simulink model "UAV_RefModel"  (R2013a)
settings: Solver=ode3  StartTime=0.0  StopTime=150  FixedStep=SampleTime  RelTol=1e-3
undefined symbols (not defined in the file or in its folder): AC, Earth, Env, IntegerTimeDelay, m, Navigation, Navigation_Lib, OperatingPoint, s, SampleTime, TrimCondition, WGS84
libraries: Sensors_Lib x13, simulink x7, aerolib6dofsys x4, Actuator_Lib x2, aerolibconvert2 x2, aerolibasang x2, aerolibutil x1, aerolibtransform2 x1, Environment_Lib x1, Aero_Lib x1, Propulsion_Lib x1, Gravity_Lib x1
settings Model: Creator=Paul Freeman  LastModifiedBy=descobar
settings DataIOCC: LimitDataPoints=off  SignalLoggingSaveFormat=ModelDataLogs  SaveOutput=off  SignalLogging=off
settings OptimizationCC: ExpressionDepthLimit=2147483647
settings DebuggingCC: FcnCallInpInsideContextMsg=UseLocalSettings  StrictBusMsg=Warning
settings HardwareCC: ProdLargestAtomicInteger=Long  ProdLargestAtomicFloat=Double  ProdIntDivRoundTo=Zero  ProdEndianess=BigEndian  ProdHWDeviceType=Freescale->32-bit PowerPC
settings SFSimCC: SimParseCustomCode=off
settings GRTTargetCC: CombineOutputUpdateFcns=off  GRTInterface=on

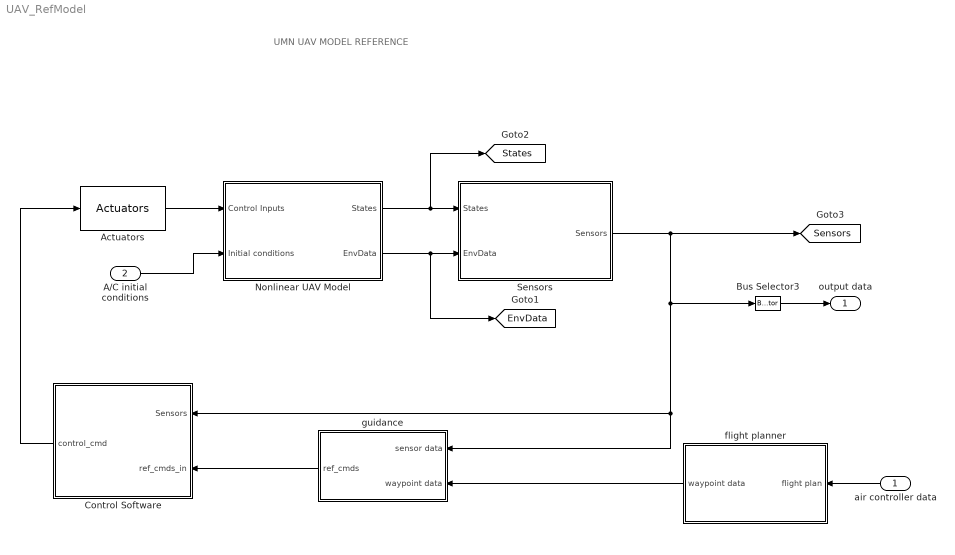
== system UAV_RefModel ==
  note: UMN UAV
      | MODEL REFERENCE
  air controller data : Inport
  A/C initial conditions : Inport  Port=2
  Actuators : Actuator_Lib/Actuators
  Bus Selector3 : BusSelector  OutputSignals=Geodetic Latitude [rad],Geodetic Longitude [rad],Altitude [m],h [m],X_e [m]  OutputAsBus=on
  Control Software : Subsystem
  Nonlinear UAV Model : Subsystem  AncestorBlock=NonlinearModel_Lib/Nonlinear UAV Model
  Sensors : Subsystem  AncestorBlock=Sensors_Lib/Sensors
  flight planner : Subsystem
  "guidance " : Subsystem
  output data : Outport
  tag scope: EnvData=global, Sensors=global, States=global
  wires:
  Sensors/1(Sensors) -> "guidance "/1(sensor data), Control Software/1(Sensors), Bus Selector3/1, [Sensors]
  Nonlinear UAV Model/1(States) -> Sensors/1(States), [States]
  Nonlinear UAV Model/2(EnvData) -> Sensors/2(EnvData), [EnvData]
  Control Software/1(control_cmd) -> Actuators/1
  Actuators/1 -> Nonlinear UAV Model/1(Control Inputs)
  "guidance "/1(ref_cmds) -> Control Software/2(ref_cmds_in)
  flight planner/1(waypoint data) -> "guidance "/2(waypoint data)
  Bus Selector3/1 -> output data/1
  air controller data/1 -> flight planner/1(flight plan)
  A/C initial conditions/1 -> Nonlinear UAV Model/2(Initial conditions)

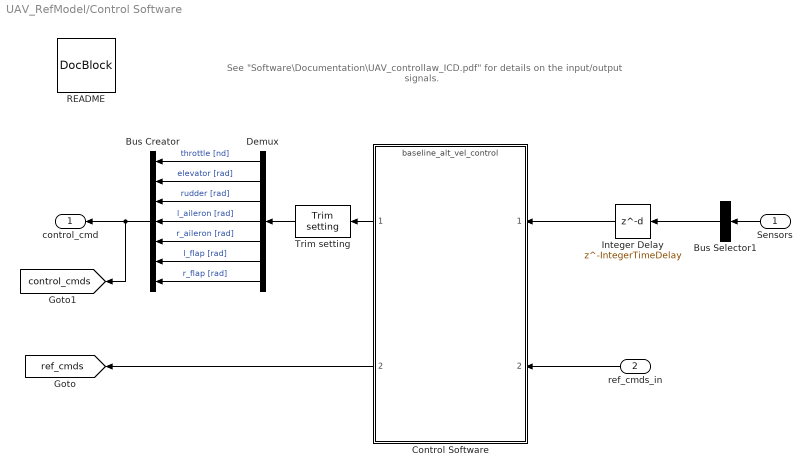
== system UAV_RefModel/Control Software ==
  note: See "Software\Documentation\UAV_controllaw_ICD.pdf" for
      | details on the input/output signals.
  Sensors : Inport
  ref_cmds_in : Inport  Port=2
  Bus Creator : BusCreator  Inputs=7
  Bus Selector1 : BusSelector  OutputSignals=phi [rad],theta [rad],psi [rad],p [rad/s],q [rad/s],r [rad/s],Ax [m/s^2],Ay [m/s^2],Az [m/s^2],h [m],V_s [m/s],alpha [rad],beta [rad],Geodetic Latitude [rad],Geodetic Longitude [rad],Altitude [m],Xdot [m/s],Ydot [m/s],Zdot [m/s]  OutputAsBus=on
  Control Software : ModelReference  ModelNameDialog=baseline_alt_vel_control  Variant=on  ModelReferenceVersion=1.189  CopyOfModelName=baseline_alt_vel_control  DefaultDataLogging=off
  Demux : Demux  Outputs=7
  Integer Delay : Delay  DelayLength=IntegerTimeDelay  InitialCondition=repmat([TrimCondition.AttitudeIni;TrimCondition.RatesIni;TrimCondition.AccelsIni;OperatingPoint.op_report.Outputs(4).y;TrimCondition.WindAxesIni;TrimCondition.LLIni;0; zeros(3,1)],[1,IntegerTimeDelay])  InputProcessing=Inherited
  README : simulink/Model-Wide Utilities/DocBlock  DocumentType=Text
      content=|
      | Control Law Block
      |
      | This block uses Model Referencing to allow the user to easily switch out
      | control law implementations. An example usage would be first a user develops
      | a control law using simulink blocks. This controller is referred to as the
      | "simulink controller" and would be selected by setting the variable
      | "controller_mode" to 2. Once the development is completed, the user then
      | implements the Simulink controller into C-code suitable for integration
      | with the UAV software. This controller is referred to as the "flight code"
      | and would be selected by setting "controller_mode" to 1.
      |
      | This is done using the Simulink.Variant object. See the documentation for
      | more detail. The user can specify any number of variants for the Control
      | Software block; edit the ModelReferenceParameters by right-clicking this
      | block to set which Simulink model is reference for each Variant object.
      | Note that these objects must be present in the base workspace. It
      | is strongly recommended that you use the "simulink_controller.mdl" file as
      | a starting place and "Save As" to a different file name.
      |
      | In summary, to switch the Control Software, modify the "contoller_mode"
      | variable:
      | 1 = flight code controller (C implementation)
      | 2 = simulink controller (empty simulink model)
      |
      |
      | See "Software\Documentation\UAV_controllaw_ICD.pdf" for details on the
      | input/output signals.
      |
      | The control_cmd signal must have the following order:
      | throttle
      | elevator
      | rudder
      | l_aileron
      | r_aileron
      | l_flap
      | r_flap
      |
      | Control Inputs Sign Convention
      | TED = Trailing Edge Down
      | TEL = Trailing Edge Left
      | ------------------------
      | Elevator: +TED
      | Rudder: +TEL
      | Aileron: +TED, da = (da_R-da_L)/2
      | Throttle: always positive
      | Flap: +TED
      |
      |
      | The refrence command signal must have the following order:
      | 1. phi_cmd
      | 2. theta_cmd
      | 3. psi_cmd
      | 4. p_cmd
      | 5. q_cmd
      | 6. r_cmd
      | 7. V_s_cmd
      | 8. h_cmd
      | 9. gndtrk_cmd
      | 10. aoa_cmd
      | 11. aos_cmd
      | 12. gamma_cmd
      | Note the trimmed value of pitch angle theta is included in the reference
      | command. Use the Doublet Generator block (or other signal generating block)
      | to input reference commands to the Control Software.
  "Trim setting " : Actuator_Lib/Trim setting 
  control_cmd : Outport
  tag scope: control_cmds=global, ref_cmds=global
  wires:
  Control Software/1 -> "Trim setting "/1
  Sensors/1 -> Bus Selector1/1
  ref_cmds_in/1 -> Control Software/2
  Bus Creator/1 -> control_cmd/1, [control_cmds]
  Demux/1 -> Bus Creator/1  "throttle [nd]"
  Demux/2 -> Bus Creator/2  "elevator [rad]"
  Demux/3 -> Bus Creator/3  "rudder [rad]"
  Demux/4 -> Bus Creator/4  "l_aileron [rad]"
  Demux/5 -> Bus Creator/5  "r_aileron [rad]"
  Demux/6 -> Bus Creator/6  "l_flap [rad]"
  Demux/7 -> Bus Creator/7  "r_flap [rad]"
  Integer Delay/1 -> Control Software/1
  Bus Selector1/1 -> Integer Delay/1
  "Trim setting "/1 -> Demux/1
  Control Software/2 -> [ref_cmds]

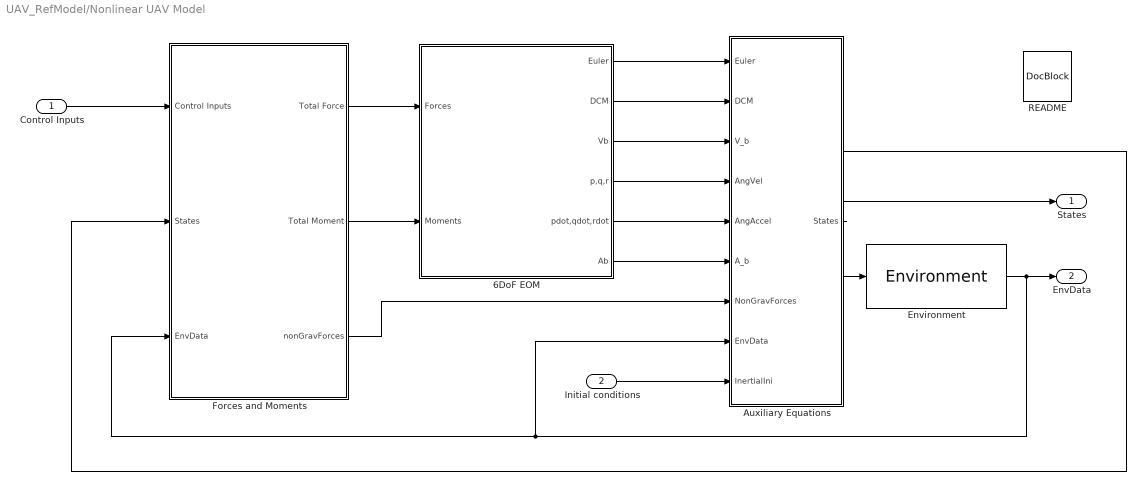
== system UAV_RefModel/Nonlinear UAV Model ==
  Control Inputs : Inport
  Initial conditions : Inport  Port=2
  6DoF EOM : Subsystem  mask(6DoF EoM (Body Axis)){units=Metric (MKS), mtype=Fixed, rep=Euler Angles, xme_0=TrimCondition.InertialIni, Vm_0=TrimCondition.VelocitiesIni, eul_0=TrimCondition.AttitudeIni, pm_0=TrimCondition.RatesIni, mass_0=AC.Mass, mass_e=0.5, mass_f=2.0, inertia=AC.Inertia.Matrix, inertia_e=eye(3), inertia_f=2*eye(3), k_quat=1.0}
      mask prompts: mtype "Mass type:"; rep "Representation:"; xme_0 "Initial position in inertial axes [Xe,Ye,Ze]:"; Vm_0 "Initial velocity in body axes [U,v,w]:"; eul_0 "Initial Euler orientation [roll, pitch, yaw]:"; pm_0 "Initial body rotation rates [p,q,r]:"; mass_0 "Initial mass:"; mass_e "Empty mass:"; mass_f "Full mass:"; inertia_e "Empty inertia matrix:"; inertia_f "Full inertia matrix:"; k_quat "Gain for quaternion normalization:"
      mask help:
      | Integrate the six-degrees-of-freedom equations of motion in body axis.
      |
      | This block has been modified from the original Aerospace Blockset
      | implementation. The inertial position vector (Xe) is no longer computed.
      | The original block did not have a way to add steady state winds to the
      | inertial velocities (Ve) prior to integrating to get Xe. Therefore, this
      | step is performed in the Auxiliary Equations block.
      mask Help: eval('asbhelp(''sixdof_euler_angles'')');
      mask TypeOptions units: Metric (MKS) | English (Velocity in ft/s) | English (Velocity in kts)
      mask TypeOptions mtype: Fixed | Simple Variable | Custom Variable
      mask Callback mtype: aeroicon('aeroblk6dofbody');
      mask TypeOptions rep: Euler Angles | Quaternion
      mask Callback rep: aeroicon('aeroblk6dofbody');
  Auxiliary Equations : Subsystem  AncestorBlock=AuxEq_Lib/Auxiliary Equations
  Environment : Environment_Lib/Environment
  Forces and Moments : Subsystem
  README : simulink/Model-Wide Utilities/DocBlock  DocumentType=Text
      content=|
      | Nonlinear UAV Model
      |
      | This block implements the nonlinear UAV dynamics model. Beginning on the
      | left, the Forces and Moments block models all of the relevant external
      | forces and moments acting on the aircraft.
      |
      | The 6DoF EOM block implements the six degree of freedom, fixed mass,
      | flat, non-rotating Earth, rigid body equations of motion. This block has
      | been modified from the original Aerospace Blockset implementation. The
      | inertial position vector (Xe) is no longer computed. The original block
      | did not have a way to add steady state winds to the inertial velocities
      | (Ve) prior to integrating to get Xe. Therefore, this step is performed in
      | the Auxiliary Equations block.
      |
      | The Auxiliary Equations computes other relevant variables (such as angle
      | of attack, indicated airspeed, etc) from state data. In this block are
      | the Navigation equations.
      |
      | Finally, the Environment block has Aerospace Blockset models for Earth's
      | atmosphere, gravity, and magnetic fields. Winds are modeled in two
      | portions: steady and unsteady. The steady portion is defined by a speed
      | and direction, and is horizontal only. The unsteady portion is made up of
      | a wind shear model and a turbulence model.
  States : Outport
  EnvData : Outport  Port=2
  wires:
  6DoF EOM/6(Ab) -> Auxiliary Equations/6(A_b)
  6DoF EOM/5(pdot,qdot,rdot) -> Auxiliary Equations/5(AngAccel)
  6DoF EOM/4(p,q,r) -> Auxiliary Equations/4(AngVel)
  6DoF EOM/3(Vb) -> Auxiliary Equations/3(V_b)
  6DoF EOM/2(DCM) -> Auxiliary Equations/2(DCM)
  6DoF EOM/1(Euler) -> Auxiliary Equations/1(Euler)
  Control Inputs/1 -> Forces and Moments/1(Control Inputs)
  Forces and Moments/1(Total Force) -> 6DoF EOM/1(Forces)
  Forces and Moments/2(Total Moment) -> 6DoF EOM/2(Moments)
  Auxiliary Equations/1(States) -> States/1, Forces and Moments/2(States), Environment/1
  Forces and Moments/3(nonGravForces) -> Auxiliary Equations/7(NonGravForces)
  Environment/1 -> Forces and Moments/3(EnvData), Auxiliary Equations/8(EnvData), EnvData/1
  Initial conditions/1 -> Auxiliary Equations/9(InertialIni)

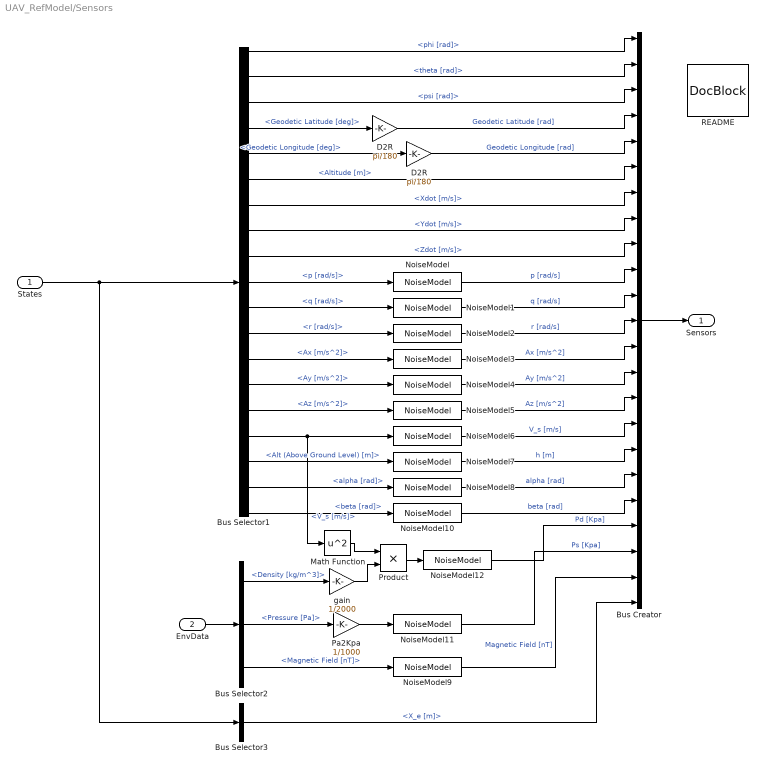
== system UAV_RefModel/Sensors ==
  States : Inport
  EnvData : Inport  Port=2
  Bus Creator : BusCreator  Inputs=23
  Bus Selector1 : BusSelector  OutputSignals=Euler [rad].phi [rad],Euler [rad].theta [rad],Euler [rad].psi [rad],Nav.Geodetic Latitude [deg],Nav.Geodetic Longitude [deg],Nav.Altitude [m],V_e [m/s].Xdot [m/s],V_e [m/s].Ydot [m/s],V_e [m/s].Zdot [m/s],AngVel [rad/s].p [rad/s],AngVel [rad/s].q [rad/s],AngVel [rad/s].r [rad/s],Accels [m/s^2].Ax [m/s^2],Accels [m/s^2].Ay [m/s^2],Accels [m/s^2].Az [m/s^2],WindAxesParam.V_s [m/s],Nav.Alt (Above Ground Level) [m],WindAxesParam.alpha [rad],WindAxesParam.beta [rad]
  Bus Selector2 : BusSelector  OutputSignals=Density [kg/m^3],Pressure [Pa],Magnetic Field [nT]
  Bus Selector3 : BusSelector  OutputSignals=X_e [m]
  D2R : Gain  Gain=pi/180  SampleTime=SampleTime
  "D2R " : Gain  Gain=pi/180  SampleTime=SampleTime
  Math Function : Math  Operator=square  SaturateOnIntegerOverflow=on
  NoiseModel : Sensors_Lib/NoiseModel  noise_on=AC.Sensors.NoiseOn  sigma=AC.Sensors.IMU.p_noise  seed=878230  bias=AC.Sensors.IMU.p_bias  scf=AC.Sensors.IMU.p_scf  timestep=SampleTime
  NoiseModel1 : Sensors_Lib/NoiseModel  noise_on=AC.Sensors.NoiseOn  sigma=AC.Sensors.IMU.q_noise  seed=878231  bias=AC.Sensors.IMU.q_bias  scf=AC.Sensors.IMU.q_scf  timestep=SampleTime
  NoiseModel10 : Sensors_Lib/NoiseModel  noise_on=AC.Sensors.NoiseOn  sigma=AC.Sensors.AirData.beta_noise  seed=87828  bias=AC.Sensors.AirData.beta_bias  scf=AC.Sensors.AirData.beta_scf  timestep=SampleTime
  NoiseModel11 : Sensors_Lib/NoiseModel  noise_on=AC.Sensors.NoiseOn  sigma=AC.Sensors.AirData.Ps_noise  seed=8782378  bias=AC.Sensors.AirData.Ps_bias  scf=AC.Sensors.AirData.Ps_scf  timestep=SampleTime
  NoiseModel12 : Sensors_Lib/NoiseModel  noise_on=AC.Sensors.NoiseOn  sigma=AC.Sensors.AirData.Pd_noise  seed=87823  bias=AC.Sensors.AirData.Pd_bias  scf=AC.Sensors.AirData.Pd_scf  timestep=SampleTime
  NoiseModel2 : Sensors_Lib/NoiseModel  noise_on=AC.Sensors.NoiseOn  sigma=AC.Sensors.IMU.r_noise  seed=878232  bias=AC.Sensors.IMU.r_bias  scf=AC.Sensors.IMU.r_scf  timestep=SampleTime
  NoiseModel3 : Sensors_Lib/NoiseModel  noise_on=AC.Sensors.NoiseOn  sigma=AC.Sensors.IMU.ax_noise  seed=878233  bias=AC.Sensors.IMU.ax_bias  scf=AC.Sensors.IMU.ax_scf  timestep=SampleTime
  NoiseModel4 : Sensors_Lib/NoiseModel  noise_on=AC.Sensors.NoiseOn  sigma=AC.Sensors.IMU.ay_noise  seed=878234  bias=AC.Sensors.IMU.ay_bias  scf=AC.Sensors.IMU.ay_scf  timestep=SampleTime
  NoiseModel5 : Sensors_Lib/NoiseModel  noise_on=AC.Sensors.NoiseOn  sigma=AC.Sensors.IMU.az_noise  seed=878235  bias=AC.Sensors.IMU.az_bias  scf=AC.Sensors.IMU.az_scf  timestep=SampleTime
  NoiseModel6 : Sensors_Lib/NoiseModel  noise_on=AC.Sensors.NoiseOn  sigma=AC.Sensors.AirData.ias_noise  seed=878236  bias=AC.Sensors.AirData.ias_bias  scf=AC.Sensors.AirData.ias_scf  timestep=SampleTime
  NoiseModel7 : Sensors_Lib/NoiseModel  noise_on=AC.Sensors.NoiseOn  sigma=AC.Sensors.AirData.h_noise  seed=87828  bias=AC.Sensors.AirData.h_bias  scf=AC.Sensors.AirData.h_scf  timestep=SampleTime
  NoiseModel8 : Sensors_Lib/NoiseModel  noise_on=AC.Sensors.NoiseOn  sigma=AC.Sensors.AirData.alpha_noise  seed=87828  bias=AC.Sensors.AirData.alpha_bias  scf=AC.Sensors.AirData.alpha_scf  timestep=SampleTime
  NoiseModel9 : Sensors_Lib/NoiseModel  noise_on=AC.Sensors.NoiseOn  sigma=[AC.Sensors.IMU.hx_noise, AC.Sensors.IMU.hy_noise,AC.Sensors.IMU.hz_noise]  seed=878237  bias=[AC.Sensors.IMU.hx_bias, AC.Sensors.IMU.hy_bias, AC.Sensors.IMU.hz_bias]  scf=[AC.Sensors.IMU.hx_scf, AC.Sensors.IMU.hy_scf, AC.Sensors.IMU.hz_scf]  timestep=SampleTime
  Pa2Kpa : Gain  Gain=1/1000
  Product : Product  RndMeth=Zero
  README : simulink/Model-Wide Utilities/DocBlock  DocumentType=Text
      content=|
      | Sensors
      |
      | This block implements sensor models on selected signals. A generic block
      | is used that applies a bias, scale factor, and band limited white noise to
      | a given signal. The parameters for each block are stored in the aircraft
      | configuration data structure (AC):
      |
      | >> AC.Sensors
      |
      | ans =
      |
      |     NoiseOn: 1
      |         IMU: [1x1 struct]
      |     AirData: [1x1 struct]
      |
      | Note the "NoiseOn" boolean flag- by setting this flag to zero, the sensor
      | model will be disabled.
      |
      | Currently, the bias and scale factor errors are not used; only white noise
      | is applied.
  gain : Gain  Gain=1/2000
  Sensors : Outport
  wires:
  Bus Selector1/15 -> NoiseModel5/1  "<Az [m/s^2]>"
  Bus Selector1/14 -> NoiseModel4/1  "<Ay [m/s^2]>"
  Bus Selector1/13 -> NoiseModel3/1  "<Ax [m/s^2]>"
  Bus Selector1/12 -> NoiseModel2/1  "<r [rad/s]>"
  Bus Selector1/11 -> NoiseModel1/1  "<q [rad/s]>"
  Bus Selector1/10 -> NoiseModel/1  "<p [rad/s]>"
  States/1 -> Bus Selector3/1, Bus Selector1/1
  Bus Selector1/16 -> NoiseModel6/1, Math Function/1  "<V_s [m/s]>"
  Bus Selector2/3 -> NoiseModel9/1  "<Magnetic Field [nT]>"
  Bus Selector1/17 -> NoiseModel7/1  "<Alt (Above Ground Level) [m]>"
  EnvData/1 -> Bus Selector2/1
  Bus Selector1/18 -> NoiseModel8/1  "<alpha [rad]>"
  Bus Selector1/19 -> NoiseModel10/1  "<beta [rad]>"
  Bus Selector2/2 -> Pa2Kpa/1  "<Pressure [Pa]>"
  Pa2Kpa/1 -> NoiseModel11/1
  Bus Selector2/1 -> gain/1  "<Density [kg/m^3]>"
  Math Function/1 -> Product/1
  gain/1 -> Product/2
  Product/1 -> NoiseModel12/1
  Bus Creator/1 -> Sensors/1
  Bus Selector1/1 -> Bus Creator/1  "<phi [rad]>"
  Bus Selector1/2 -> Bus Creator/2  "<theta [rad]>"
  Bus Selector1/3 -> Bus Creator/3  "<psi [rad]>"
  Bus Selector1/4 -> D2R/1  "<Geodetic Latitude [deg]>"
  Bus Selector1/5 -> "D2R "/1  "<Geodetic Longitude [deg]>"
  Bus Selector1/6 -> Bus Creator/6  "<Altitude [m]>"
  Bus Selector1/7 -> Bus Creator/7  "<Xdot [m/s]>"
  Bus Selector1/8 -> Bus Creator/8  "<Ydot [m/s]>"
  Bus Selector1/9 -> Bus Creator/9  "<Zdot [m/s]>"
  NoiseModel/1 -> Bus Creator/10  "p [rad/s]"
  NoiseModel1/1 -> Bus Creator/11  "q [rad/s]"
  NoiseModel2/1 -> Bus Creator/12  "r [rad/s]"
  NoiseModel3/1 -> Bus Creator/13  "Ax [m/s^2]"
  NoiseModel4/1 -> Bus Creator/14  "Ay [m/s^2]"
  NoiseModel5/1 -> Bus Creator/15  "Az [m/s^2]"
  NoiseModel6/1 -> Bus Creator/16  "V_s [m/s]"
  NoiseModel7/1 -> Bus Creator/17  "h [m]"
  NoiseModel8/1 -> Bus Creator/18  "alpha [rad]"
  NoiseModel10/1 -> Bus Creator/19  "beta [rad]"
  NoiseModel12/1 -> Bus Creator/20  "Pd [Kpa]"
  NoiseModel11/1 -> Bus Creator/21  "Ps [Kpa]"
  NoiseModel9/1 -> Bus Creator/22  "Magnetic Field [nT]"
  D2R/1 -> Bus Creator/4  "Geodetic Latitude [rad]"
  "D2R "/1 -> Bus Creator/5  "Geodetic Longitude [rad]"
  Bus Selector3/1 -> Bus Creator/23  "<X_e [m]>"

== system UAV_RefModel/flight planner ==
  flight plan : Inport
  Bus Creator : BusCreator  Inputs=2
  Waypoint generator : MATLAB Function  TreatAsAtomicUnit=on
  waypoint data : Outport
  wires:
  Waypoint generator/1(waypoint) -> Bus Creator/1
  Waypoint generator/2(nPoints) -> Bus Creator/2
  Bus Creator/1 -> waypoint data/1
  flight plan/1 -> Waypoint generator/1(plan)

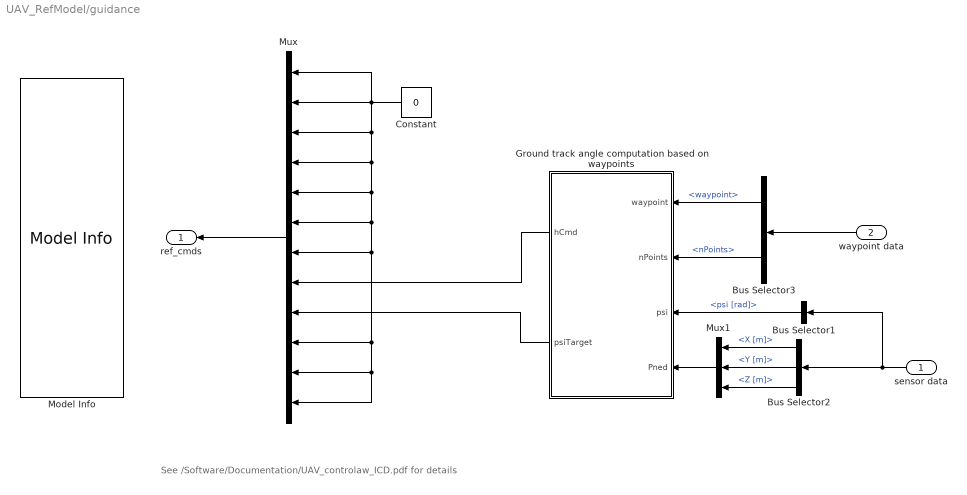
== system UAV_RefModel/guidance  ==
  note: See /Software/Documentation/UAV_controlaw_ICD.pdf
      | for details
  sensor data : Inport
  waypoint data : Inport  Port=2
  Bus Selector1 : BusSelector  OutputSignals=psi [rad]
  Bus Selector2 : BusSelector  OutputSignals=X_e [m].X [m],X_e [m].Y [m],X_e [m].Z [m]
  Bus Selector3 : BusSelector  OutputSignals=waypoint,nPoints
  Constant : Constant  Value=0
  Ground track angle computation based on waypoints : MATLAB Function  TreatAsAtomicUnit=on
  Model Info : simulink/Model-Wide Utilities/Model Info  InitialBlockCM=None  BlockCM=None  Frame=on  DisplayStringWithTags=|  HorizontalTextAlignment=Center  LeftAlignmentValue=0.5  SourceBlockDiagram=UAV_RefModel  TagMaxNumber=20
      | Ref Cmd Port Info
      | 
      | 1. phi_cmd
      | 2. theta_cmd
      | 3. psi_cmd
      | 4. p_cmd
      | 5. q_cmd
      | 6. r_cmd
      | 7. V_s_cmd
      | 8. h_cmd
      | 9. gndtrk_cmd
      | 10. aoa_cmd
      | 11. aos_cmd
      | 12. gamma_cmd
  Mux : Mux  Inputs=12
  Mux1 : Mux  Inputs=3
  ref_cmds : Outport
  wires:
  Mux/1 -> ref_cmds/1
  Bus Selector2/1 -> Mux1/1  "<X [m]>"
  Bus Selector2/2 -> Mux1/2  "<Y [m]>"
  Bus Selector2/3 -> Mux1/3  "<Z [m]>"
  sensor data/1 -> Bus Selector1/1, Bus Selector2/1
  Bus Selector1/1 -> Ground track angle computation based on waypoints/3(psi)  "<psi [rad]>"
  Mux1/1 -> Ground track angle computation based on waypoints/4(Pned)
  Bus Selector3/1 -> Ground track angle computation based on waypoints/1(waypoint)  "<waypoint>"
  Bus Selector3/2 -> Ground track angle computation based on waypoints/2(nPoints)  "<nPoints>"
  Ground track angle computation based on waypoints/2(psiTarget) -> Mux/9
  Constant/1 -> Mux/3, Mux/4, Mux/5, Mux/6, Mux/7, Mux/10, Mux/11, Mux/12, Mux/1, Mux/2
  waypoint data/1 -> Bus Selector3/1
  Ground track angle computation based on waypoints/1(hCmd) -> Mux/8

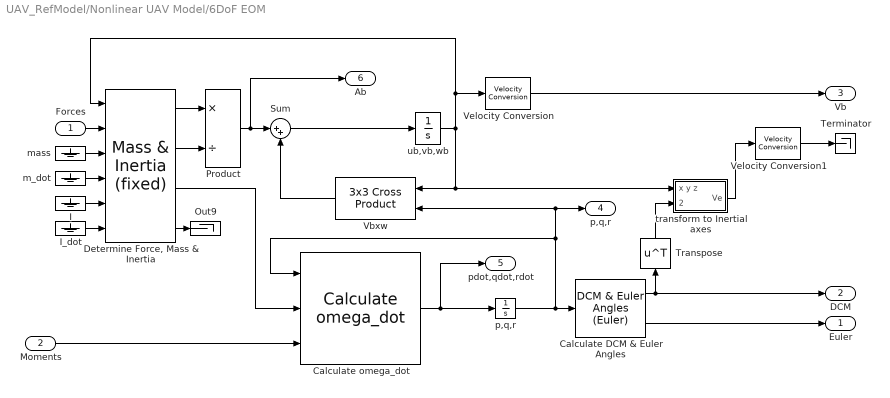
== system UAV_RefModel/Nonlinear UAV Model/6DoF EOM ==
  Forces : Inport
  Moments : Inport  Port=2
  Calculate DCM & Euler Angles : aerolib6dofsys/DCM & Euler Angles (Euler)  SystemSampleTime=-1
  Calculate omega_dot : aerolib6dofsys/Calculate omega_dot
  "Determine Force, Mass & Inertia" : aerolib6dofsys/Mass & Inertia (fixed)  SystemSampleTime=-1
  I : Ground
  I_dot : Ground
  Out9 : Terminator
  Product : Product  Inputs=*/  SaturateOnIntegerOverflow=on  OutDataTypeStr=Inherit: Same as first input
  Sum : Sum  Inputs=|++  SaturateOnIntegerOverflow=on
  Terminator : Terminator
  Transpose : Math  Operator=transpose  SaturateOnIntegerOverflow=on
  Vbxw : aerolibutil/3x3 Cross Product
  Velocity Conversion : aerolibconvert2/Velocity Conversion  IU=m/s  OU=m/s
  Velocity Conversion1 : aerolibconvert2/Velocity Conversion  IU=m/s  OU=m/s
  m_dot : Ground
  mass : Ground
  "p,q,r " : Integrator  InitialCondition=pm_0
  "transform to Inertial axes " : Subsystem  mask(Vector Transformation){}
      mask Display: disp('L_EB')
  ub,vb,wb : Integrator  InitialCondition=convvel(Vm_0,'m/s','m/s')
  Euler : Outport
  DCM : Outport  Port=2
  Vb : Outport  Port=3
  p,q,r : Outport  Port=4
  pdot,qdot,rdot : Outport  Port=5
  Ab : Outport  Port=6
  wires:
  Velocity Conversion1/1 -> Terminator/1
  Velocity Conversion/1 -> Vb/1
  "Determine Force, Mass & Inertia"/3 -> Calculate omega_dot/2
  Calculate DCM & Euler Angles/2 -> Euler/1
  Vbxw/1 -> Sum/2
  ub,vb,wb/1 -> Velocity Conversion/1, "Determine Force, Mass & Inertia"/1, "transform to Inertial axes "/1(x y z), Vbxw/1
  Sum/1 -> ub,vb,wb/1
  "transform to Inertial axes "/1(Ve) -> Velocity Conversion1/1
  "p,q,r "/1 -> Calculate omega_dot/1, p,q,r/1, Vbxw/2, Calculate DCM & Euler Angles/1
  Moments/1 -> Calculate omega_dot/3
  Forces/1 -> "Determine Force, Mass & Inertia"/2
  Product/1 -> Sum/1, Ab/1
  Calculate DCM & Euler Angles/1 -> DCM/1, Transpose/1
  Transpose/1 -> "transform to Inertial axes "/2(transform coefficients)
  mass/1 -> "Determine Force, Mass & Inertia"/3
  "Determine Force, Mass & Inertia"/2 -> Product/2
  m_dot/1 -> "Determine Force, Mass & Inertia"/4
  "Determine Force, Mass & Inertia"/4 -> Out9/1
  Calculate omega_dot/1 -> pdot,qdot,rdot/1, "p,q,r "/1
  I/1 -> "Determine Force, Mass & Inertia"/5
  I_dot/1 -> "Determine Force, Mass & Inertia"/6
  "Determine Force, Mass & Inertia"/1 -> Product/1

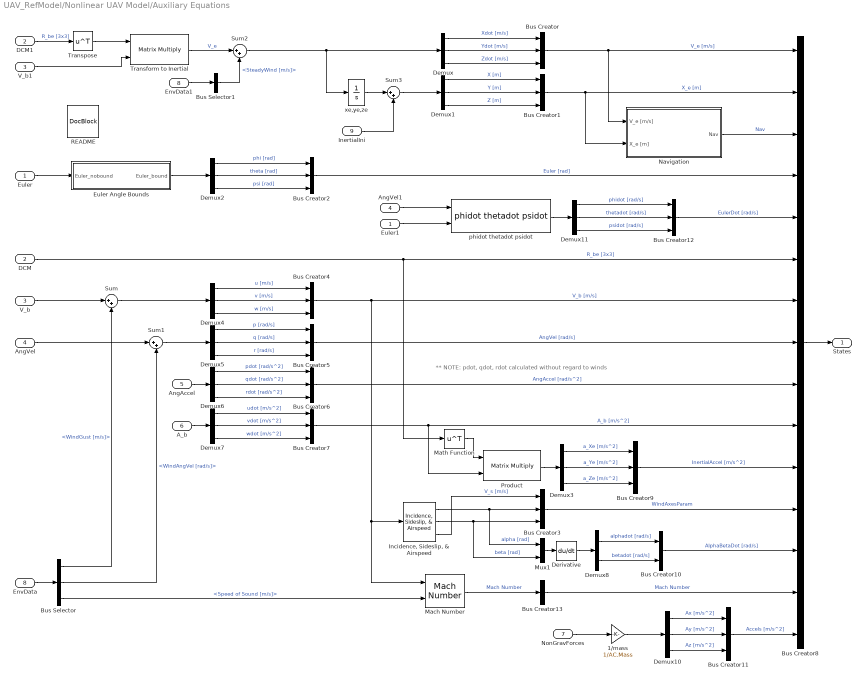
== system UAV_RefModel/Nonlinear UAV Model/Auxiliary Equations ==
  note: ** NOTE: pdot, qdot, rdot calculated without regard to winds
  Euler : Inport
  DCM : Inport  Port=2
  V_b : Inport  Port=3
  AngVel : Inport  Port=4
  AngAccel : Inport  Port=5
  A_b : Inport  Port=6
  NonGravForces : Inport  Port=7
  EnvData : Inport  Port=8
  InertialIni : Inport  Port=9
  1/mass : Gain  Gain=1/AC.Mass
  AngVel1 : InportShadow  Port=4
  Bus Creator{,1..7,9,11..12} (11 alike) : BusCreator  Inputs=3
  Bus Creator10 : BusCreator  Inputs=2
  Bus Creator13 : BusCreator  Inputs=1
  Bus Creator8 : BusCreator  Inputs=15
  Bus Selector : BusSelector  OutputSignals=WindGust [m/s],WindAngVel [rad/s],Speed of Sound [m/s]
  Bus Selector1 : BusSelector  OutputSignals=SteadyWind [m/s]
  DCM1 : InportShadow  Port=2
  Demux{,1..7,10..11} (10 alike) : Demux  Outputs=3
  Demux8 : Demux  Outputs=2
  Derivative : Derivative
  EnvData1 : InportShadow  Port=8
  Euler Angle Bounds : Subsystem
  Euler1 : InportShadow
  "Incidence, Sideslip, & Airspeed" : aerolibasang/Incidence, Sideslip, & Airspeed
  Mach Number : aerolibasang/Mach Number
  Math Function : Math  Operator=transpose  SaturateOnIntegerOverflow=on
  Mux1 : Mux  Inputs=2
  Navigation : Subsystem  Description=|  AncestorBlock=Navigation_Lib/Navigation
      | This model produces the followng navigation data for the UAV flight:
      |                                                                     
      | * Geodetic Latitude                                                 
      | * Geodetic Longitude                                                
      | * Geodetic Altitude                                                 
      | * Altitude above Mean Sea Level                                     
      | * Gravitational acceleration vector
  Product : Product  Multiplication=Matrix(*)  RndMeth=Zero
  README : simulink/Model-Wide Utilities/DocBlock  DocumentType=Text
      content=|
      | Auxiliary Equations
      |
      | This block computes other relevant variables (such as angle of attack,
      | indicated airspeed, etc) from state data. Part of this block is simply to
      | assign signals name and create the States bus.
      |
      | Working from the top of the block downwards:
      |
      | The inertial velocity, V_e, is computed by using the Direction Cosine
      | Matrix (DCM) to transform the body-axis velocities (u,v,w) to the
      | inertial frame. The steady state winds are then added, and the result is
      | V_e. This is integrated to obtain the inertial position, X_e.  The
      | initial condition of the X_e integrator is set by
      | TrimCondition.InertialIni. V_e and X_e are inputs to the Navigation
      | block- see that blocks README for details.
      |
      | Euler angles are bounded by +\- [pi/2, pi, 2*pi] respectively. The time
      | derivatives of the Euler angles are computed using the body-axis rates
      | and the Euler angles.
      |
      | The DCM is included in the States bus as "R_be [3x3]".
      |
      | Body axis velocites and rates, and their derivatives are included. The
      | unsteady (turbulence and gusts) winds are added to the body axis
      | velocities and rates.
      |
      | Inertial accelerations are computed by transforming the body-axis
      | accelerations with the DCM. This step is simplified since we are using a
      | non-rotating Earth.
      |
      | WindAxesParam is the true airspeed, angle of attack, and sideslip angle.
      | The derivatives of alpha and beta are computed using a deriative block.
      | Mach number is simply the ratio between true airspeed and the speed of
      | sound.
      |
      | Accels [m/s^2] is what an accelerometer would read onboard the aircraft.
      |
      | *Note on winds: dividing the wind components into steady and unsteady
      | components is necessary because we do not use an intermediate atmospheric
      | reference frame to account for the motion of the air mass relative to the
      | Earth. We can approximate the physical effects of wind without an
      | additional reference frame by splitting the wind into steady and unsteady
      | components, where the steady component is added to the inertial
      | velocities and the unsteady component is added to the body-axis
      | velocities allows us to
  Sum{,1..3} (4 alike) : Sum  Inputs=|++
  Transform to Inertial : Product  Multiplication=Matrix(*)  RndMeth=Zero
  Transpose : Math  Operator=transpose  SaturateOnIntegerOverflow=on
  V_b1 : InportShadow  Port=3
  phidot thetadot psidot : aerolib6dofsys/DCM & Euler Angles (Euler)/phidot thetadot psidot
  xe,ye,ze : Integrator  InitialCondition=TrimCondition.InertialIni
  States : Outport
  wires:
  Mach Number/1 -> Bus Creator13/1  "Mach Number"
  Demux8/2 -> Bus Creator10/2  "betadot [rad/s]"
  Demux8/1 -> Bus Creator10/1  "alphadot [rad/s]"
  Bus Creator10/1 -> Bus Creator8/13  "AlphaBetaDot [rad/s]"
  Derivative/1 -> Demux8/1
  Mux1/1 -> Derivative/1
  "Incidence, Sideslip, & Airspeed"/3 -> Bus Creator3/1  "V_s [m/s]"
  "Incidence, Sideslip, & Airspeed"/2 -> Mux1/2, Bus Creator3/3  "beta [rad]"
  "Incidence, Sideslip, & Airspeed"/1 -> Mux1/1, Bus Creator3/2  "alpha [rad]"
  Bus Creator8/1 -> States/1
  Navigation/1(Nav) -> Bus Creator8/3  "Nav"
  Bus Creator11/1 -> Bus Creator8/15  "Accels [m/s^2]"
  Euler1/1 -> phidot thetadot psidot/2
  AngVel1/1 -> phidot thetadot psidot/1
  Bus Selector/1 -> Sum/2  "<WindGust [m/s]>"
  Bus Selector/2 -> Sum1/2  "<WindAngVel [rad/s]>"
  Bus Creator9/1 -> Bus Creator8/11  "InertialAccel [m/s^2]"
  Demux3/2 -> Bus Creator9/2  "a_Ye [m/s^2]"
  Demux3/3 -> Bus Creator9/3  "a_Ze [m/s^2]"
  Demux3/1 -> Bus Creator9/1  "a_Xe [m/s^2]"
  Product/1 -> Demux3/1
  Math Function/1 -> Product/1
  V_b/1 -> Sum/1
  AngVel/1 -> Sum1/1
  Sum/1 -> Demux4/1
  Sum1/1 -> Demux5/1
  Bus Selector/3 -> Mach Number/2  "<Speed of Sound [m/s]>"
  EnvData/1 -> Bus Selector/1
  Bus Creator13/1 -> Bus Creator8/14  "Mach Number"
  Bus Creator3/1 -> Bus Creator8/12  "WindAxesParam"
  A_b/1 -> Demux7/1
  Demux7/3 -> Bus Creator7/3  "wdot [m/s^2]"
  Demux7/2 -> Bus Creator7/2  "vdot [m/s^2]"
  Demux7/1 -> Bus Creator7/1  "udot [m/s^2]"
  Bus Creator7/1 -> Bus Creator8/10, Product/2  "A_b [m/s^2]"
  AngAccel/1 -> Demux6/1
  Demux6/3 -> Bus Creator6/3  "rdot [rad/s^2]"
  Demux6/2 -> Bus Creator6/2  "qdot [rad/s^2]"
  Demux6/1 -> Bus Creator6/1  "pdot [rad/s^2]"
  Bus Creator6/1 -> Bus Creator8/9  "AngAccel [rad/s^2]"
  Demux5/3 -> Bus Creator5/3  "r [rad/s]"
  Demux5/2 -> Bus Creator5/2  "q [rad/s]"
  Demux5/1 -> Bus Creator5/1  "p [rad/s]"
  Bus Creator5/1 -> Bus Creator8/8  "AngVel [rad/s]"
  Demux4/3 -> Bus Creator4/3  "w [m/s]"
  Demux4/2 -> Bus Creator4/2  "v [m/s]"
  Demux4/1 -> Bus Creator4/1  "u [m/s]"
  Bus Creator4/1 -> Mach Number/1, "Incidence, Sideslip, & Airspeed"/1, Bus Creator8/7  "V_b [m/s]"
  DCM/1 -> Bus Creator8/6, Math Function/1  "R_be [3x3]"
  Demux2/3 -> Bus Creator2/3  "psi [rad]"
  Demux2/2 -> Bus Creator2/2  "theta [rad]"
  Demux2/1 -> Bus Creator2/1  "phi [rad]"
  Bus Creator2/1 -> Bus Creator8/4  "Euler [rad]"
  Demux1/3 -> Bus Creator1/3  "Z [m]"
  Demux1/2 -> Bus Creator1/2  "Y [m]"
  Demux1/1 -> Bus Creator1/1  "X [m]"
  Bus Creator1/1 -> Bus Creator8/2, Navigation/2(X_e [m])  "X_e [m]"
  Demux/3 -> Bus Creator/3  "Zdot [m/s]"
  Demux/2 -> Bus Creator/2  "Ydot [m/s]"
  Demux/1 -> Bus Creator/1  "Xdot [m/s]"
  Bus Creator/1 -> Bus Creator8/1, Navigation/1(V_e [m/s])  "V_e [m/s]"
  NonGravForces/1 -> 1/mass/1
  1/mass/1 -> Demux10/1
  Demux10/1 -> Bus Creator11/1  "Ax [m/s^2]"
  Demux10/2 -> Bus Creator11/2  "Ay [m/s^2]"
  Demux10/3 -> Bus Creator11/3  "Az [m/s^2]"
  Demux11/3 -> Bus Creator12/3  "psidot [rad/s]"
  Demux11/2 -> Bus Creator12/2  "thetadot [rad/s]"
  Demux11/1 -> Bus Creator12/1  "phidot [rad/s]"
  Bus Creator12/1 -> Bus Creator8/5  "EulerDot [rad/s]"
  phidot thetadot psidot/1 -> Demux11/1
  Transpose/1 -> Transform to Inertial/1
  DCM1/1 -> Transpose/1  "R_be [3x3]"
  EnvData1/1 -> Bus Selector1/1
  Transform to Inertial/1 -> Sum2/1  "V_e"
  Bus Selector1/1 -> Sum2/2  "<SteadyWind [m/s]>"
  Sum2/1 -> Demux/1, xe,ye,ze/1
  V_b1/1 -> Transform to Inertial/2
  Euler/1 -> Euler Angle Bounds/1(Euler_nobound)
  Euler Angle Bounds/1(Euler_bound) -> Demux2/1
  Sum3/1 -> Demux1/1
  xe,ye,ze/1 -> Sum3/1
  InertialIni/1 -> Sum3/2

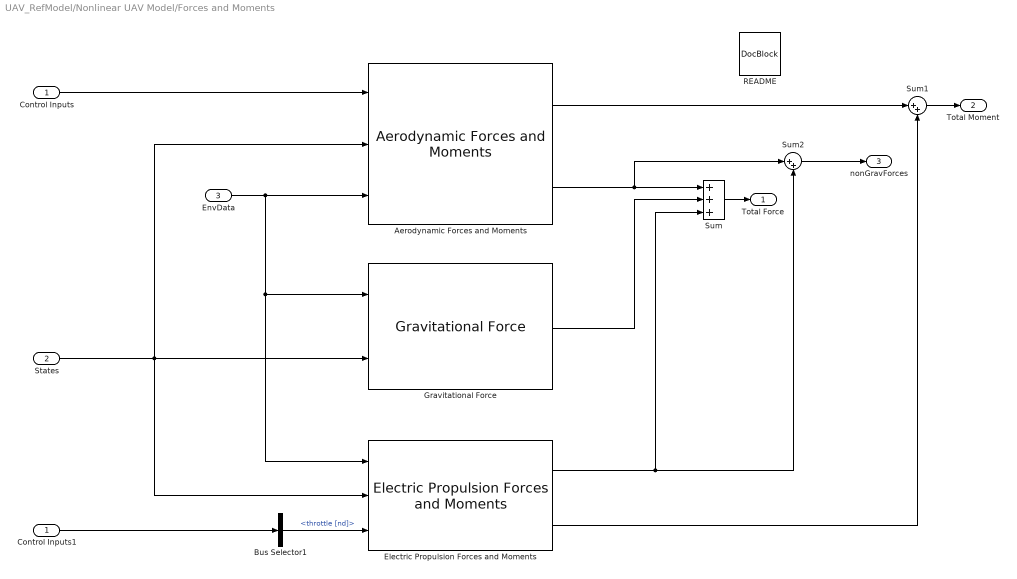
== system UAV_RefModel/Nonlinear UAV Model/Forces and Moments ==
  Control Inputs : Inport
  States : Inport  Port=2
  EnvData : Inport  Port=3
  Aerodynamic Forces and Moments : Aero_Lib/Aerodynamic Forces and Moments  aeromodel=AC.Aero.use_FASER_aero
  Bus Selector1 : BusSelector  OutputSignals=throttle [nd]
  Control Inputs1 : InportShadow
  Electric Propulsion Forces and Moments : Propulsion_Lib/Electric Propulsion Forces and Moments
  "Gravitational Force " : Gravity_Lib/Gravitational Force 
  README : simulink/Model-Wide Utilities/DocBlock  DocumentType=Text
      content=|
      | Forces and Moments
      |
      | This block models all of the relevant external forces and
      | moments acting on the aircraft. The Aerodynamic Forces and Moments block
      | contains the aero models, and is a masked subsystem. The input parameter to
      | this block is a boolean which controls which aero model (either FASER or
      | the Ultrastick) is used.
      |
      | The Gravitational Force block models the effect of Earth's graviy field on
      | the aircraft.
      |
      | The Electric Propulsion Forces and Moments block contains the electric
      | motor model.
      |
      | Note the non-gravitational forces (nonGravForces) are output- this is what
      | an accelerometer on the aircraft would measure, and is used in the sensor
      | models.
  Sum : Sum  Inputs=+++
  Sum1 : Sum  Inputs=|++
  Sum2 : Sum  Inputs=|++
  Total Force : Outport
  Total Moment : Outport  Port=2
  nonGravForces : Outport  Port=3
  wires:
  Bus Selector1/1 -> Electric Propulsion Forces and Moments/3  "<throttle [nd]>"
  Control Inputs/1 -> Aerodynamic Forces and Moments/1
  States/1 -> Aerodynamic Forces and Moments/2, "Gravitational Force "/2, Electric Propulsion Forces and Moments/2
  EnvData/1 -> Aerodynamic Forces and Moments/3, "Gravitational Force "/1, Electric Propulsion Forces and Moments/1
  Control Inputs1/1 -> Bus Selector1/1
  Aerodynamic Forces and Moments/2 -> Sum/1, Sum2/1
  "Gravitational Force "/1 -> Sum/2
  Electric Propulsion Forces and Moments/1 -> Sum2/2, Sum/3
  Sum/1 -> Total Force/1
  Aerodynamic Forces and Moments/1 -> Sum1/1
  Electric Propulsion Forces and Moments/2 -> Sum1/2
  Sum1/1 -> Total Moment/1
  Sum2/1 -> nonGravForces/1

== system UAV_RefModel/Nonlinear UAV Model/6DoF EOM/transform to Inertial axes  ==
  x y z : Inport
  transform coefficients : Inport  Port=2
  Product : Product  Multiplication=Matrix(*)  SaturateOnIntegerOverflow=on  InputSameDT=on  OutDataTypeStr=Inherit: Same as first input
  Reshape1 : Reshape  OutputDimensionality=Column vector (2-D)
  Reshape2 : Reshape
  Ve : Outport
  wires:
  Product/1 -> Reshape2/1
  transform coefficients/1 -> Product/1
  x y z/1 -> Reshape1/1
  Reshape1/1 -> Product/2
  Reshape2/1 -> Ve/1

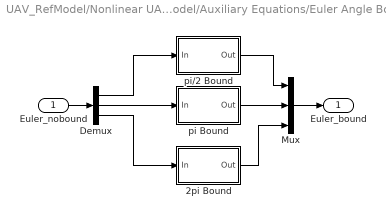
== system UAV_RefModel/Nonlinear UAV Model/Auxiliary Equations/Euler Angle Bounds ==
  Euler_nobound : Inport
  2pi Bound : Subsystem
  Demux : Demux  Outputs=3
  Mux : Mux  Inputs=3
  pi Bound : Subsystem
  pi/2 Bound : Subsystem
  Euler_bound : Outport
  wires:
  2pi Bound/1(Out) -> Mux/3
  Demux/3 -> 2pi Bound/1(In)
  Demux/2 -> pi Bound/1(In)
  Demux/1 -> pi/2 Bound/1(In)
  Euler_nobound/1 -> Demux/1
  Mux/1 -> Euler_bound/1
  pi/2 Bound/1(Out) -> Mux/1
  pi Bound/1(Out) -> Mux/2

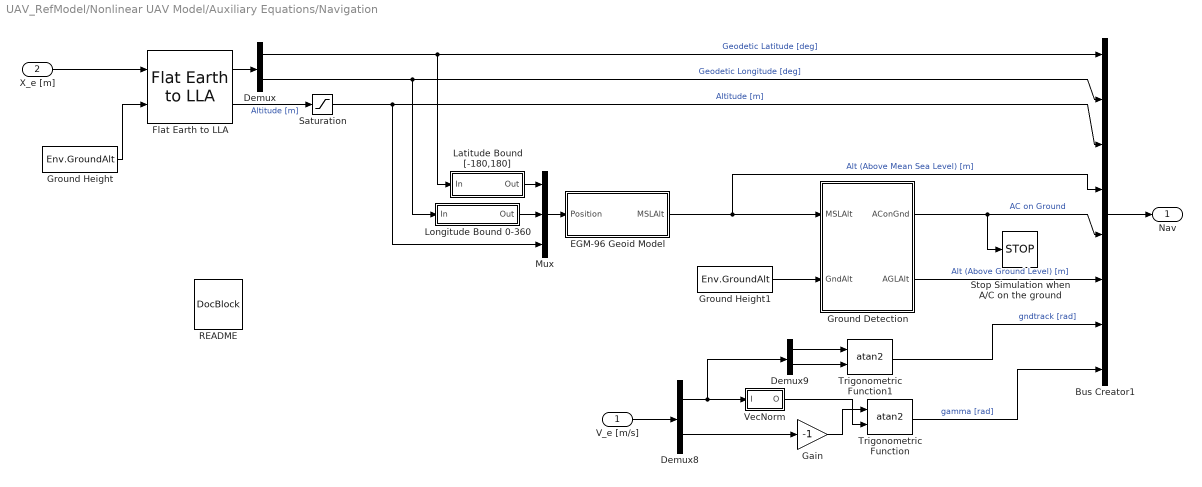
== system UAV_RefModel/Nonlinear UAV Model/Auxiliary Equations/Navigation ==
  V_e [m/s] : Inport
  X_e [m] : Inport  Port=2
  Bus Creator1 : BusCreator  Inputs=8
  Demux : Demux  Outputs=2
  Demux8 : Demux  Outputs=[2 1]
  Demux9 : Demux  Outputs=2
  EGM-96 Geoid Model : Subsystem  mask(EGM-96 geoid undulation model){}
      mask help: Computes the MSL (mean sea level) altitude as a function of position.
      mask init:
      | load('egm96');
      mask Help:
      | The block computes the mean-sea-level altitude relative to the WGS-84 geoid.
      | <P><B>Inputs:</B>
      | <LI>Position = the 3x1 vector of aircraft location [Latitude Longitude Altitude], in [rad rad m]</LI>
      | </P>
      | <P><B>Output:</B>
      | <LI>MSLAlt = the mean-sea-level altitude, in m</LI>
      | </P>
  Flat Earth to LLA : aerolibtransform2/Flat Earth to LLA  units=Metric (MKS)  ptype=Earth (WGS84)  F=1/298.257223563  R=6378137  LL0=TrimCondition.LLIni  psi=0
  Gain : Gain  Gain=-1
  Ground Detection : Subsystem  mask(Ground detection){}
      mask help: Computes altitude above ground and sets a flag if AGL is negative.
      mask Help:
      | The block computes the altitude above ground (AGL) and sets a flag if the AGL is negative (used for ground contact detection).
      | <P><B>Inputs:</B>
      | <LI>MSLAlt = the altitude measured from mean-sea-level, in meters</LI>
      | <LI>GndAlt = the altitude of the terrain (above MSL) at current location, in meters</LI>
      | </P>
      | <P><B>Output:</B>
      | <LI>AConGnd = the aircraft-on-ground flag (0 if aircraft above ground, 1 if aircraft on the ground)</LI>
      | <LI>AGLAlt = the altitude of the aircraft above ground</LI>
      | </P>
  Ground Height : Constant  Value=Env.GroundAlt
  Ground Height1 : Constant  Value=Env.GroundAlt
  Latitude Bound [-180,180] : Subsystem
  Longitude Bound 0-360 : Subsystem  mask(Longitude bound){}
      mask help: Bounds the longitude to [0, 2pi]. When 0 bound is exceeded the longitude wraps back to 2pi; when the 2pi bound is exceeded the longitude wraps back to 0.
  Mux : Mux  Inputs=3
  README : simulink/Model-Wide Utilities/DocBlock  DocumentType=Text
      content=|
      | Navigation
      |
      | This block is library link that contains the navigational model and
      | equations. Included are equations relating the flat Earth position to
      | latitude/longitude, a simplified 2D table lookup version of the EGM-96
      | Geoid model for computation of MSL/AGL altitudes, and computation of
      | flight path and ground track angles.
  Saturation : Saturate  UpperLimit=Inf  LowerLimit=0
  Stop Simulation when A/C on the ground : Stop
  Trigonometric Function : Trigonometry  Operator=atan2
  Trigonometric Function1 : Trigonometry  Operator=atan2
  VecNorm : Subsystem
  Nav : Outport
  wires:
  Gain/1 -> Trigonometric Function/1
  Latitude Bound [-180,180]/1(Out) -> Mux/1
  Longitude Bound 0-360/1(Out) -> Mux/2
  Demux9/1 -> Trigonometric Function1/1
  Demux8/1 -> Demux9/1, VecNorm/1(I)
  Trigonometric Function1/1 -> Bus Creator1/7  "gndtrack [rad]"
  Demux9/2 -> Trigonometric Function1/2
  Trigonometric Function/1 -> Bus Creator1/8  "gamma [rad]"
  VecNorm/1(O) -> Trigonometric Function/2
  Demux8/2 -> Gain/1
  V_e [m/s]/1 -> Demux8/1
  Ground Detection/2(AGLAlt) -> Bus Creator1/6  "Alt (Above Ground Level) [m]"
  Mux/1 -> EGM-96 Geoid Model/1(Position)
  Saturation/1 -> Mux/3, Bus Creator1/3  "Altitude [m]"
  Ground Detection/1(AConGnd) -> Bus Creator1/5, Stop Simulation when A/C on the ground/1  "AC on Ground"
  Ground Height1/1 -> Ground Detection/2(GndAlt)
  EGM-96 Geoid Model/1(MSLAlt) -> Ground Detection/1(MSLAlt), Bus Creator1/4  "Alt (Above Mean Sea Level) [m]"
  Bus Creator1/1 -> Nav/1
  Ground Height/1 -> Flat Earth to LLA/2
  X_e [m]/1 -> Flat Earth to LLA/1
  Demux/2 -> Longitude Bound 0-360/1(In), Bus Creator1/2  "Geodetic Longitude [deg]"
  Demux/1 -> Latitude Bound [-180,180]/1(In), Bus Creator1/1  "Geodetic Latitude [deg]"
  Flat Earth to LLA/2 -> Saturation/1  "Altitude [m]"
  Flat Earth to LLA/1 -> Demux/1

== system UAV_RefModel/Nonlinear UAV Model/Auxiliary Equations/Euler Angle Bounds/2pi Bound ==
  In : Inport
  2pi : Constant  Value=2*pi
  Math Function : Math  Operator=mod  SaturateOnIntegerOverflow=on
  Out : Outport
  wires:
  In/1 -> Math Function/1
  2pi/1 -> Math Function/2
  Math Function/1 -> Out/1

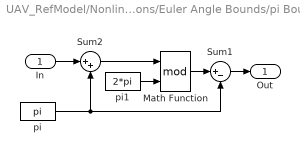
== system UAV_RefModel/Nonlinear UAV Model/Auxiliary Equations/Euler Angle Bounds/pi Bound ==
  In : Inport
  Math Function : Math  Operator=mod  SaturateOnIntegerOverflow=on
  Sum1 : Sum  Inputs=|+-  SaturateOnIntegerOverflow=on  InputSameDT=on  OutDataTypeStr=Inherit: Same as first input
  Sum2 : Sum  Inputs=|++  SaturateOnIntegerOverflow=on  InputSameDT=on  OutDataTypeStr=Inherit: Same as first input
  pi : Constant  Value=pi
  pi1 : Constant  Value=2*pi
  Out : Outport
  wires:
  Sum1/1 -> Out/1
  pi/1 -> Sum1/2, Sum2/2
  Sum2/1 -> Math Function/1
  In/1 -> Sum2/1
  pi1/1 -> Math Function/2
  Math Function/1 -> Sum1/1

== system UAV_RefModel/Nonlinear UAV Model/Auxiliary Equations/Euler Angle Bounds/pi//2 Bound ==
  In : Inport
  Math Function : Math  Operator=mod  SaturateOnIntegerOverflow=on
  Sum1 : Sum  Inputs=|+-  SaturateOnIntegerOverflow=on  InputSameDT=on  OutDataTypeStr=Inherit: Same as first input
  Sum2 : Sum  Inputs=|++  SaturateOnIntegerOverflow=on  InputSameDT=on  OutDataTypeStr=Inherit: Same as first input
  pi : Constant  Value=pi/2
  pi1 : Constant  Value=pi
  Out : Outport
  wires:
  Math Function/1 -> Sum1/1
  pi1/1 -> Math Function/2
  In/1 -> Sum2/1
  Sum2/1 -> Math Function/1
  pi/1 -> Sum2/2, Sum1/2
  Sum1/1 -> Out/1

== system UAV_RefModel/Nonlinear UAV Model/Auxiliary Equations/Navigation/EGM-96 Geoid Model ==
  Position : Inport
  Demux2 : Demux  Outputs=3
  Look-Up Table (2-D) : Lookup2D  RowIndex=Lat  ColumnIndex=Lon  Table=Alterr'  SaturateOnIntegerOverflow=on  InputSameDT=on
  Sum : Sum  Inputs=|+++
  WGS-84 correction : Constant  Value=-0.53
  MSLAlt : Outport
  wires:
  WGS-84 correction/1 -> Sum/3
  Look-Up Table (2-D)/1 -> Sum/1
  Sum/1 -> MSLAlt/1
  Demux2/3 -> Sum/2
  Position/1 -> Demux2/1
  Demux2/1 -> Look-Up Table (2-D)/1
  Demux2/2 -> Look-Up Table (2-D)/2

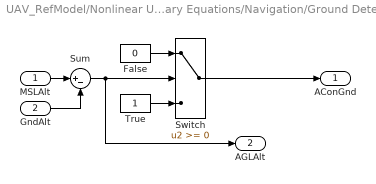
== system UAV_RefModel/Nonlinear UAV Model/Auxiliary Equations/Navigation/Ground Detection ==
  MSLAlt : Inport
  GndAlt : Inport  Port=2
  False : Constant  Value=0
  Sum : Sum  Inputs=|+-  SaturateOnIntegerOverflow=on  InputSameDT=on  OutDataTypeStr=Inherit: Same as first input
  Switch : Switch  SaturateOnIntegerOverflow=on  InputSameDT=on
  True : Constant
  AConGnd : Outport
  AGLAlt : Outport  Port=2
  wires:
  MSLAlt/1 -> Sum/1
  GndAlt/1 -> Sum/2
  Sum/1 -> Switch/2, AGLAlt/1
  False/1 -> Switch/1
  True/1 -> Switch/3
  Switch/1 -> AConGnd/1

== system UAV_RefModel/Nonlinear UAV Model/Auxiliary Equations/Navigation/Latitude Bound [-180,180] ==
  In : Inport
  2pi : Constant  Value=360
  Math Function : Math  Operator=mod  SaturateOnIntegerOverflow=on
  Sum1 : Sum  Inputs=|+-  SaturateOnIntegerOverflow=on  InputSameDT=on  OutDataTypeStr=Inherit: Same as first input
  Sum2 : Sum  Inputs=|++  SaturateOnIntegerOverflow=on  InputSameDT=on  OutDataTypeStr=Inherit: Same as first input
  pi : Constant  Value=180
  Out : Outport
  wires:
  Math Function/1 -> Sum1/1
  2pi/1 -> Math Function/2
  In/1 -> Sum2/1
  Sum2/1 -> Math Function/1
  pi/1 -> Sum2/2, Sum1/2
  Sum1/1 -> Out/1

== system UAV_RefModel/Nonlinear UAV Model/Auxiliary Equations/Navigation/Longitude Bound 0-360 ==
  In : Inport
  2pi : Constant  Value=360
  Math Function : Math  Operator=mod  SaturateOnIntegerOverflow=on
  Out : Outport
  wires:
  Math Function/1 -> Out/1
  2pi/1 -> Math Function/2
  In/1 -> Math Function/1

== system UAV_RefModel/Nonlinear UAV Model/Auxiliary Equations/Navigation/VecNorm ==
  I : Inport
  Math Function2 : Math  Operator=sqrt  SaturateOnIntegerOverflow=on
  Product : Product  RndMeth=Zero
  Sum of Elements : Sum  Inputs=+
  O : Outport
  wires:
  Sum of Elements/1 -> Math Function2/1
  Product/1 -> Sum of Elements/1
  I/1 -> Product/2, Product/1
  Math Function2/1 -> O/1

== matlab function UAV_RefModel/guidance /Ground track angle computation based on waypoints ==
  data: hCmd output; waypoint input; nPoints input; psi input; Pned input; psiTarget output
function [hCmd ,psiTarget]     = fcn(waypoint, nPoints, psi, Pned )
%#codegen
psiErrorMax = 90*pi/180; 
RTurnMin = 150; 

hCmd = 0;

% persitent variable used to keep trak of next waypoint
persistent wpointer; 

% persitent variable used to keep track of operation mode. 
% mode = 1: tracking next waypoint
% mode = 2: tracking an intermediate waypoint to guarantee 
persistent mode; 

% auxilary waypoint coordinates for operation in mode 2
persistent wpointAux; 

if isempty(wpointer) 
wpointer = 1; 
end

if isempty(mode) 
mode = 1; 
end

if isempty(wpointAux) 
wpointAux = zeros(2, 2);  
end

psiTarget =0;

% a waypoint is reached if the distance to the aircraft is less than 20 m
if (mode ==1 && norm(Pned(1:2) - waypoint(:, wpointer) )< 10 ) 
    if(wpointer ~= nPoints)        
      
        psiTarget = atan2( waypoint(2,wpointer+1) - Pned(2) , waypoint(1,wpointer+1) - Pned(1)) ;
        % psiTarget from 0 to 360 deg only
        if (psiTarget <0)
            psiTarget = 2*pi+psiTarget ; 
        end
        
        psiError = psiTarget - psi; 
        
        if (psiError > psiErrorMax)
            mode = 2;
            % after intermediate waypoint we will pass through the last
            % waypoint

            psiAux = psiTarget - pi; 
            wpointAux(1,1) = Pned(1)+  RTurnMin*cos(psiAux) ; 
            wpointAux(2,1) = Pned(2)+  RTurnMin*sin(psiAux) ; 
            
            wpointAux(1,2) = Pned(1)+  RTurnMin*cos(psiAux)/2 ; 
            wpointAux(2,2) = Pned(2)+  RTurnMin*sin(psiAux)/2 ; 
            
            disp('aus wpoint')
            wpointAux
            disp('my pos')
            Pned(1:2)
            
            disp('psi trget')
            psiTarget
            
            
            
        else
            wpointer = wpointer + 1 
        end

        %{
        if (psiError < -pi)
            psiError = 2*pi+psiError ; 
        end

        if (psiError > pi)
            psiError = -2*pi+psiError ; 
        end
        %}
        
    end
    
    
end

if (mode ==2 && norm(Pned(1:2) - wpointAux (:,1) )< 10)

    mode =3 ; 
    
    disp('aux mode 2 completed')
end

if (mode ==3 && norm(Pned(1:2) - wpointAux (:,2) )< 10)

    mode =1 ; 
    
    disp('aux mode 3 completed')
end


if mode ==1 
% computing the angle between the vehicle ground velocity vector and vector
% connecting thevehicle body frame and waypoint
psiTarget = atan2( waypoint(2,wpointer) - Pned(2) , waypoint(1,wpointer) - Pned(1)) ;
end

if mode ==2
  psiTarget = atan2( wpointAux(2,1) - Pned(2) , wpointAux(1,1) - Pned(1)) ;
end

if mode ==3
  psiTarget = atan2( wpointAux(2,2) - Pned(2) , wpointAux(1,2) - Pned(1)) ;
end


% psiTarget from 0 to 360 deg only
if (psiTarget <0)
    psiTarget = 2*pi+psiTarget ; 
end

== matlab function UAV_RefModel/flight planner/Waypoint generator ==
  data: waypoint output; nPoints output; plan input
function [waypoint, nPoints]  = fcn (plan)
%#codegen

nPoints = 10; 

waypoint = zeros(2,nPoints);

waypoint(:,1) = [-200; 80] ; 

waypoint(:,2) = [-400; 100] ; 

waypoint(:,3) = [-600; 100] ; 

waypoint(:,4) = [-800; 300] ; 

waypoint(:,5) = [-1200; 180] ; 

waypoint(:,6) = [-1200; -180] ; 

waypoint(:,7) = [-800; -300] ; 

waypoint(:,8) = [-600; -100] ; 

waypoint(:,9) = [-400; -100] ; 

waypoint(:,10) = [-200; -80] ;
